simulink model "XInput_Controller_SFun_Builder"  (R2019a)
settings: Solver=VariableStepAuto  StartTime=0.0  StopTime=inf  RelTol=1e-3
settings Model: Creator=Mathias Voigt  LastModifiedBy=Mathias Voigt

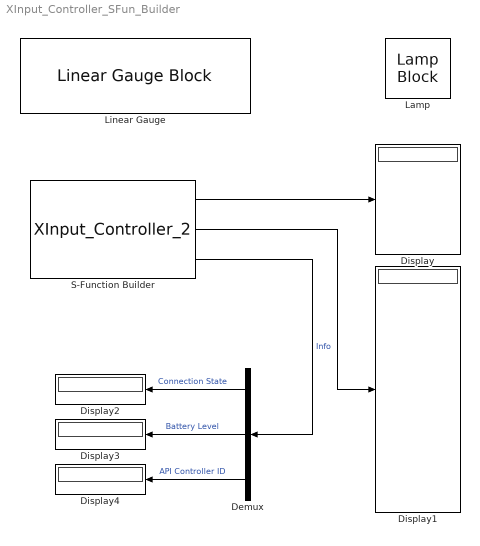
== system XInput_Controller_SFun_Builder ==
  Demux : Demux  Outputs=3
  Display{,1..4} (5 alike) : Display
  Lamp : LampBlock
  Linear Gauge : LinearGaugeBlock  TickInterval=25
  S-Function Builder : S-Function  InitFcn=try, set_param(gcb,'FunctionName','XInput_Controller_2'), end  FunctionName=XInput_Controller_2  Parameters=1  SFunctionModules=XInput_Controller_2_wrapper  SFunctionDeploymentMode=off  EnableBusSupport=off  mask(S-Function Builder){}
      mask help: Simulink:masks:SFunctionBuilder_MD
      mask init:
      | val = [[.9  0.75 0.75 1 1 .9 .9 1]',[1 1 0.75 0.75 .9 .9 1 .9]'];try , sys = get_param(gcb,'SfunBuilderFcnName');if isempty(sys), sys = get_param(gcb,'FunctionName'); end,catch, sys = get_param(gcb,'FunctionName'); end
      settings: CopyFcn=set_param(gcbh,'LinkStatus','none')  PreSaveFcn=try, set_param(gcb,'FunctionName','XInput_Controller_2'), end  OpenFcn=sfunctionwizard(gcbh)
      mask Display: plot(val(:,1),val(:,2)),disp(sys), port_label('output',1,'axes'), port_label('output',2,'buttons'), port_label('output',3,'info')
  wires:
  Demux/2 -> Display3/1  "Battery Level"
  Demux/3 -> Display4/1  "API Controller ID"
  Demux/1 -> Display2/1  "Connection State"
  S-Function Builder/3 -> Demux/1  "Info"
  S-Function Builder/2 -> Display1/1
  S-Function Builder/1 -> Display/1
